simulink model "Exp3_FT"  (R2023a)
settings: Solver=ode4  StartTime=0.0  StopTime=10.0  FixedStep=0.01  RelTol=1e-3
undefined symbols (not defined in the file): A, B, C, D, d1, G1, G2, G3, G4, G5, n1
settings Model: Creator=carlo  LastModifiedBy=carlo

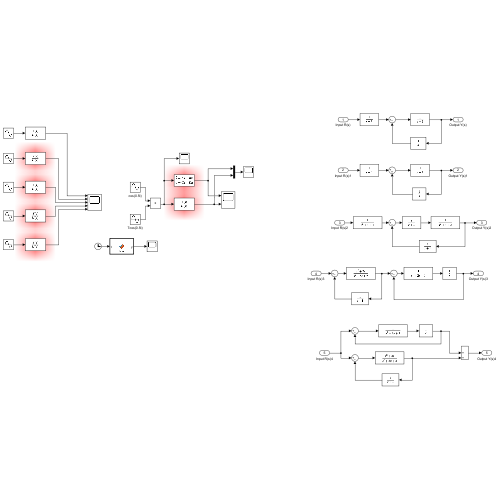
[thumbnail: Simulink's stored preview of the top-level diagram]
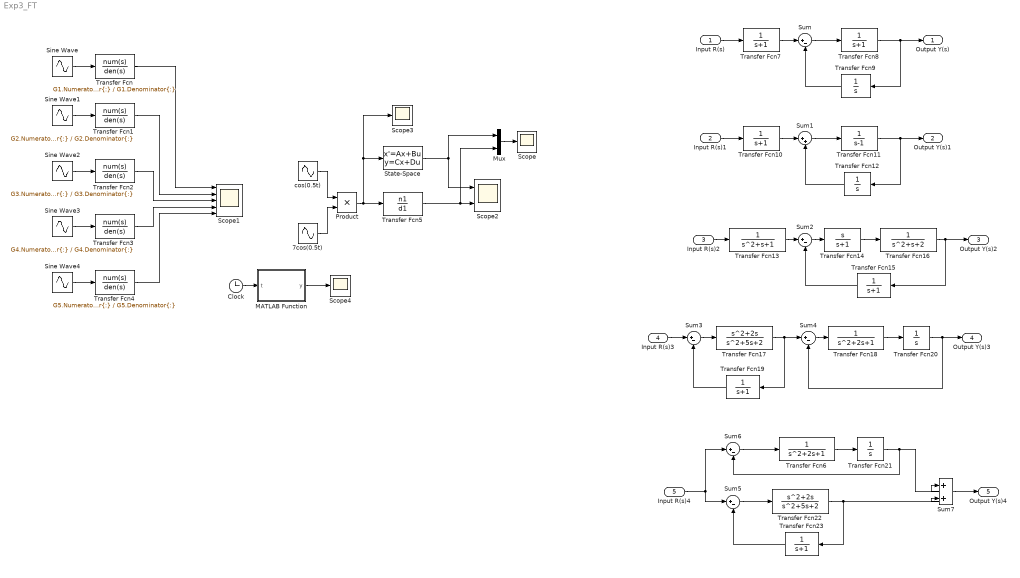
== system Exp3_FT ==
  Input R(s) : Inport
  Input R(s)1 : Inport  Port=2
  Input R(s)2 : Inport  Port=3
  Input R(s)3 : Inport  Port=4
  Input R(s)4 : Inport  Port=5
  7cos(0.5t) : Sin  Amplitude=7  Frequency=0.5  Phase=pi/2  SampleTime=0
  Clock : Clock
  MATLAB Function : MATLAB Function  TreatAsAtomicUnit=on
  Mux : Mux  Inputs=2
  Product : Product
  Scope : Scope
  Scope1 : Scope  NumInputPorts=5
  Scope2 : Scope  NumInputPorts=2
  Scope3 : Scope
  Scope4 : Scope
  Sine Wave{,1..4} (5 alike) : Sin  Frequency=2  SampleTime=0
  State-Space : StateSpace  A=A  B=B  C=C  D=D  InitialCondition=[0;0;0]
  Sum{,2..6} (6 alike) : Sum  Inputs=|+-
  Sum1 : Sum  Inputs=|++
  Sum7 : Sum  Inputs=|++
  Transfer Fcn : TransferFcn  Numerator=G1.Numerator{:}  Denominator=G1.Denominator{:}
  Transfer Fcn1 : TransferFcn  Numerator=G2.Numerator{:}  Denominator=G2.Denominator{:}
  Transfer Fcn{7..8,10,15,19,23} (6 alike) : TransferFcn  Denominator=[1 1]
  Transfer Fcn11 : TransferFcn  Denominator=[1 -1]
  Transfer Fcn{9,12,20..21} (4 alike) : TransferFcn  Denominator=[1 0]
  Transfer Fcn13 : TransferFcn  Denominator=[1 1 1]
  Transfer Fcn14 : TransferFcn  Numerator=[1 0]  Denominator=[1 1]
  Transfer Fcn16 : TransferFcn  Denominator=[1 1 2]
  Transfer Fcn17 : TransferFcn  Numerator=[1 2 0]  Denominator=[1 5 2]
  Transfer Fcn18 : TransferFcn
  Transfer Fcn2 : TransferFcn  Numerator=G3.Numerator{:}  Denominator=G3.Denominator{:}
  Transfer Fcn22 : TransferFcn  Numerator=[1 2 0]  Denominator=[1 5 2]
  Transfer Fcn3 : TransferFcn  Numerator=G4.Numerator{:}  Denominator=G4.Denominator{:}
  Transfer Fcn4 : TransferFcn  Numerator=G5.Numerator{:}  Denominator=G5.Denominator{:}
  Transfer Fcn5 : TransferFcn  Numerator=n1  Denominator=d1
  Transfer Fcn6 : TransferFcn
  cos(0.5t) : Sin  Frequency=0.5  Phase=pi/2  SampleTime=0
  Output Y(s) : Outport
  Output Y(s)1 : Outport  Port=2
  Output Y(s)2 : Outport  Port=3
  Output Y(s)3 : Outport  Port=4
  Output Y(s)4 : Outport  Port=5
  wires:
  Sine Wave/1 -> Transfer Fcn/1
  Sine Wave1/1 -> Transfer Fcn1/1
  Sine Wave2/1 -> Transfer Fcn2/1
  Sine Wave3/1 -> Transfer Fcn3/1
  Sine Wave4/1 -> Transfer Fcn4/1
  Transfer Fcn/1 -> Scope1/1
  Transfer Fcn1/1 -> Scope1/2
  Transfer Fcn2/1 -> Scope1/3
  Transfer Fcn3/1 -> Scope1/4
  Transfer Fcn4/1 -> Scope1/5
  cos(0.5t)/1 -> Product/1
  7cos(0.5t)/1 -> Product/2
  Product/1 -> State-Space/1, Scope3/1, Transfer Fcn5/1
  Transfer Fcn5/1 -> Mux/2, Scope2/2
  State-Space/1 -> Scope2/1, Mux/1
  Mux/1 -> Scope/1
  Clock/1 -> MATLAB Function/1(t)
  MATLAB Function/1(y) -> Scope4/1
  Transfer Fcn8/1 -> Transfer Fcn9/1, Output Y(s)/1
  Input R(s)/1 -> Transfer Fcn7/1
  Transfer Fcn9/1 -> Sum/2
  Transfer Fcn7/1 -> Sum/1
  Sum/1 -> Transfer Fcn8/1
  Sum1/1 -> Transfer Fcn11/1
  Transfer Fcn10/1 -> Sum1/1
  Transfer Fcn12/1 -> Sum1/2
  Input R(s)1/1 -> Transfer Fcn10/1
  Transfer Fcn11/1 -> Output Y(s)1/1, Transfer Fcn12/1
  Transfer Fcn14/1 -> Transfer Fcn16/1
  Input R(s)2/1 -> Transfer Fcn13/1
  Transfer Fcn15/1 -> Sum2/2
  Transfer Fcn13/1 -> Sum2/1
  Sum2/1 -> Transfer Fcn14/1
  Transfer Fcn16/1 -> Transfer Fcn15/1, Output Y(s)2/1
  Transfer Fcn18/1 -> Transfer Fcn20/1
  Input R(s)3/1 -> Sum3/1
  Sum3/1 -> Transfer Fcn17/1
  Transfer Fcn19/1 -> Sum3/2
  Transfer Fcn17/1 -> Transfer Fcn19/1, Sum4/1
  Sum4/1 -> Transfer Fcn18/1
  Transfer Fcn20/1 -> Output Y(s)3/1, Sum4/2
  Input R(s)4/1 -> Sum6/1, Sum5/1
  Sum6/1 -> Transfer Fcn6/1
  Transfer Fcn6/1 -> Transfer Fcn21/1
  Sum5/1 -> Transfer Fcn22/1
  Transfer Fcn23/1 -> Sum5/2
  Transfer Fcn22/1 -> Transfer Fcn23/1, Sum7/2
  Sum7/1 -> Output Y(s)4/1
  Transfer Fcn21/1 -> Sum6/2, Sum7/1

== matlab function Exp3_FT/MATLAB Function ==
  data: t input; y output
function y = fcn(t)

y = 7*(cos(0.5*t))^2;
